simulink model "lookupTableDynamic_TestGen27"  (R2017b)
settings: Solver=FixedStepDiscrete  StartTime=0.0  StopTime=10.0  RelTol=1e-3
libraries: simulink x1
settings Model: Creator=ktrinh  LastModifiedBy=ktrinh
settings DebuggingCC: ParameterOverflowMsg=none

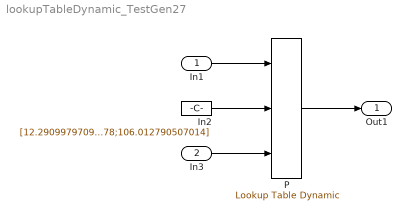
== system lookupTableDynamic_TestGen27 ==
  In1 : Inport  OutMin=10.291  OutMax=108  OutDataTypeStr=int8  PortDimensions=[2,3]
  In3 : Inport  Port=2  PortDimensions=5
  In2 : Constant  Value=[12.2909979709469;51.0837557988449;81.986279708065;99.6211568255078;106.012790507014]  OutDataTypeStr=int8
  P : simulink/Lookup Tables/Lookup Table Dynamic  LookUpMeth=Use Input Below  OutDataType=fixdt('double')  OutScaling=2^-10  OutDataTypeStr=Inherit: Inherit via back propagation  RndMeth=Zero  DoSatur=on
      settings: SourceProductName=Simulink
  Out1 : Outport
  wires:
  In1/1 -> P/1
  In2/1 -> P/2
  In3/1 -> P/3
  P/1 -> Out1/1
